simulink model "quad_modelling"  (R2015a)
settings: Solver=ode45  StartTime=0.0  StopTime=10.0  RelTol=1e-3
settings Model: Creator=USER  LastModifiedBy=USER

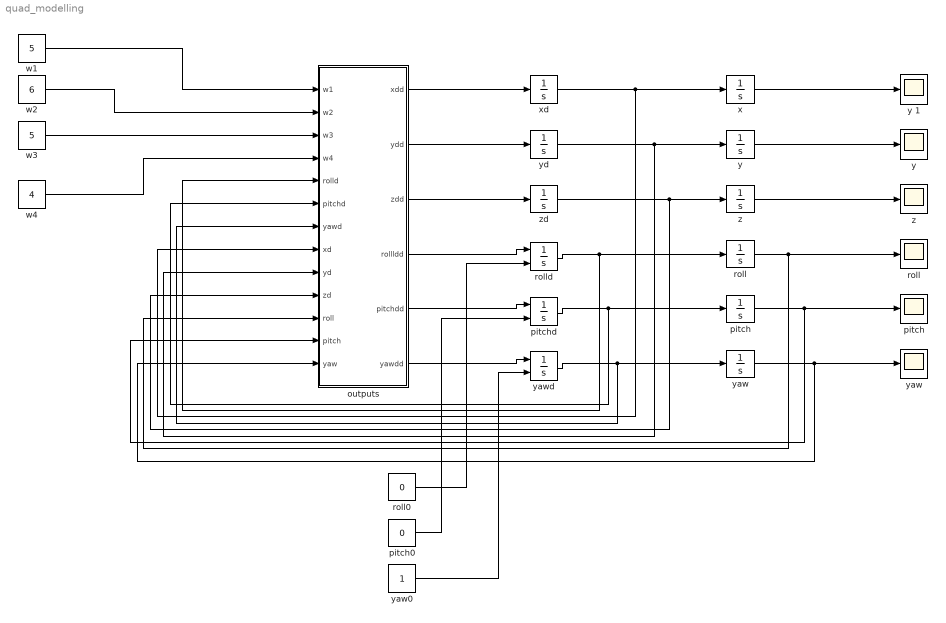
== system quad_modelling ==
  outputs : Subsystem
  pitch : Integrator
  "pitch " : Scope
  pitch0 : Constant  Value=0
  pitchd : Integrator  InitialConditionSource=external
  roll : Integrator
  "roll " : Scope
  roll0 : Constant  Value=0
  rolld : Integrator  InitialConditionSource=external
  w1 : Constant  Value=5
  w2 : Constant  Value=6
  w3 : Constant  Value=5
  w4 : Constant  Value=4
  x : Integrator
  xd : Integrator
  y : Integrator
  "y " : Scope
      settings: TimeRange=10  YMin=0  YMax=400  SaveName=ScopeData5
  y 1 : Scope
      settings: TimeRange=10  YMin=0  YMax=400  SaveName=ScopeData6
  yaw : Integrator
  "yaw " : Scope
      settings: YMin=3.125  YMax=3.35  SaveName=ScopeData2
  yaw0 : Constant
  yawd : Integrator  InitialConditionSource=external
  yd : Integrator
  z : Integrator
  "z " : Scope
      settings: TimeRange=10  YMin=7.7  YMax=8.3  SaveName=ScopeData3
  zd : Integrator
  wires:
  outputs/4(rollldd) -> rolld/1
  outputs/5(pitchdd) -> pitchd/1
  pitchd/1 -> outputs/6("pitchd "), pitch/1
  outputs/6(yawdd) -> yawd/1
  yawd/1 -> outputs/7(yawd), yaw/1
  roll/1 -> outputs/11(roll), "roll "/1
  pitch/1 -> outputs/12(pitch), "pitch "/1
  yaw/1 -> outputs/13(yaw), "yaw "/1
  w1/1 -> outputs/1("w1 ")
  w2/1 -> outputs/2("w2 ")
  w3/1 -> outputs/3("w3 ")
  outputs/3("zdd ") -> zd/1
  zd/1 -> outputs/10(zd), z/1
  z/1 -> "z "/1
  w4/1 -> outputs/4("w4 ")
  outputs/1("xdd ") -> xd/1
  outputs/2("ydd ") -> yd/1
  yd/1 -> outputs/9(yd), y/1
  x/1 -> y 1/1
  y/1 -> "y "/1
  rolld/1 -> outputs/5("rolld "), roll/1
  xd/1 -> outputs/8(xd), x/1
  roll0/1 -> rolld/2
  pitch0/1 -> pitchd/2
  yaw0/1 -> yawd/2

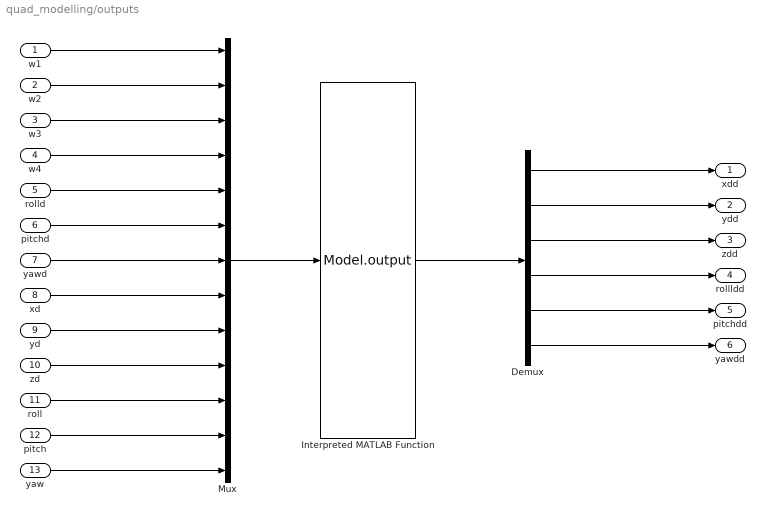
== system quad_modelling/outputs ==
  "w1 " : Inport
  "w2 " : Inport  Port=2
  "w3 " : Inport  Port=3
  "w4 " : Inport  Port=4
  "rolld " : Inport  Port=5
  "pitchd " : Inport  Port=6
  yawd : Inport  Port=7
  xd : Inport  Port=8
  yd : Inport  Port=9
  zd : Inport  Port=10
  roll : Inport  Port=11
  pitch : Inport  Port=12
  yaw : Inport  Port=13
  Demux : Demux  Outputs=6
  Interpreted MATLAB Function : MATLABFcn  MATLABFcn=Model.output  OutputDimensions=6
  Mux : Mux  Inputs=13
  "xdd " : Outport
  "ydd " : Outport  Port=2
  "zdd " : Outport  Port=3
  rollldd : Outport  Port=4
  pitchdd : Outport  Port=5
  yawdd : Outport  Port=6
  wires:
  "w1 "/1 -> Mux/1
  "w2 "/1 -> Mux/2
  "w3 "/1 -> Mux/3
  Interpreted MATLAB Function/1 -> Demux/1
  Demux/4 -> rollldd/1
  Demux/5 -> pitchdd/1
  Demux/6 -> yawdd/1
  Mux/1 -> Interpreted MATLAB Function/1
  "pitchd "/1 -> Mux/6
  "rolld "/1 -> Mux/5
  "w4 "/1 -> Mux/4
  yawd/1 -> Mux/7
  xd/1 -> Mux/8
  yd/1 -> Mux/9
  zd/1 -> Mux/10
  Demux/1 -> "xdd "/1
  roll/1 -> Mux/11
  pitch/1 -> Mux/12
  yaw/1 -> Mux/13
  Demux/2 -> "ydd "/1
  Demux/3 -> "zdd "/1
